simulink library "ECO_TestLibs"  (R2018a)
settings: Solver=ode45  StartTime=0.0  StopTime=10.0  RelTol=1e-3  EnableMultiTasking=on
undefined symbols (not defined in the file or in its folder): h, km
libraries: CoderSF_BSW_Libs x643, $bdroot x217, SF_CanService_Libs x60, simulink x12
(part 3 of 7)

== system ECO_TestLibs/TAF_CAND/Enabled Subsystem ==
  In1 : Inport
  Enable : EnablePort
  "Send CAN Message " : SF_CanService_Libs/Send CAN Message   typeCAN=Connected  channel=CAN_D  mEn=off  msgInfo=TAF_CAN_new  msgIterm=CAN0x7fc  msgItermStore=CAN0x7fc  motoBit=off  flgNoFixed=off  tSample=Task_MDef  modeCode=Parameterless
  Send CAN Message 1 : SF_CanService_Libs/Send CAN Message   typeCAN=Connected  channel=CAN_D  mEn=off  msgInfo=TAF_CAN_new  msgIterm=CAN0x1ffffffc  msgItermStore=CAN0x1ffffffc  motoBit=off  flgNoFixed=off  tSample=Task_MDef  modeCode=Parameterless
  wires:
  In1/1 -> Send CAN Message 1/1, "Send CAN Message "/1

== system ECO_TestLibs/TAF_CAND/Receive CAN Message ==
  Receive CAN Message : CoderSF_BSW_Libs/CAN/Receive CAN Message  channel=CAN_D  txid=hex2dec('100')  extended=off  txlen=8  tasktimeIndex=Task_L1ms
      settings: SourceProductName=EcoCoder Blocks
  Receive CAN Message1 : CoderSF_BSW_Libs/CAN/Receive CAN Message  channel=CAN_D  txid=hex2dec('100')  extended=off  txlen=8  tasktimeIndex=Task_L1ms
      settings: SourceProductName=EcoCoder Blocks
  Receive CAN Message2 : CoderSF_BSW_Libs/CAN/Receive CAN Message  channel=CAN_D  txid=hex2dec('100')  extended=off  txlen=8  tasktimeIndex=Task_L1ms
      settings: SourceProductName=EcoCoder Blocks
  Write Measurement1 : CoderSF_BSW_Libs/Calibration & Measurement/Write Measurement  variable_name=CANDR1_flgAvailable  variable_value=0  variable_type=boolean  numD=1  unitStr=""  descStr=""
      settings: AttributesFormatString=type:%<variable_type> Dimensions:%<numD>  SourceProductName=EcoCoder Blocks
  Write Measurement10 : CoderSF_BSW_Libs/Calibration & Measurement/Write Measurement  variable_name=CANDR2_id  variable_value=0  variable_type=uint32  numD=1  unitStr=""  descStr=""
      settings: AttributesFormatString=type:%<variable_type> Dimensions:%<numD>  SourceProductName=EcoCoder Blocks
  Write Measurement11 : CoderSF_BSW_Libs/Calibration & Measurement/Write Measurement  variable_name=CANDR2_len  variable_value=0  variable_type=uint8  numD=1  unitStr=""  descStr=""
      settings: AttributesFormatString=type:%<variable_type> Dimensions:%<numD>  SourceProductName=EcoCoder Blocks
  Write Measurement12 : CoderSF_BSW_Libs/Calibration & Measurement/Write Measurement  variable_name=CANDR2_data  variable_value=0  variable_type=uint8  numD=8  unitStr=""  descStr=""
      settings: AttributesFormatString=type:%<variable_type> Dimensions:%<numD>  SourceProductName=EcoCoder Blocks
  Write Measurement13 : CoderSF_BSW_Libs/Calibration & Measurement/Write Measurement  variable_name=CANDR3_id  variable_value=0  variable_type=uint32  numD=1  unitStr=""  descStr=""
      settings: AttributesFormatString=type:%<variable_type> Dimensions:%<numD>  SourceProductName=EcoCoder Blocks
  Write Measurement14 : CoderSF_BSW_Libs/Calibration & Measurement/Write Measurement  variable_name=CANDR3_len  variable_value=0  variable_type=uint8  numD=1  unitStr=""  descStr=""
      settings: AttributesFormatString=type:%<variable_type> Dimensions:%<numD>  SourceProductName=EcoCoder Blocks
  Write Measurement15 : CoderSF_BSW_Libs/Calibration & Measurement/Write Measurement  variable_name=CANDR3_data  variable_value=0  variable_type=uint8  numD=8  unitStr=""  descStr=""
      settings: AttributesFormatString=type:%<variable_type> Dimensions:%<numD>  SourceProductName=EcoCoder Blocks
  Write Measurement16 : CoderSF_BSW_Libs/Calibration & Measurement/Write Measurement  variable_name=CANDR3_flgAvailable  variable_value=0  variable_type=boolean  numD=1  unitStr=""  descStr=""
      settings: AttributesFormatString=type:%<variable_type> Dimensions:%<numD>  SourceProductName=EcoCoder Blocks
  Write Measurement17 : CoderSF_BSW_Libs/Calibration & Measurement/Write Measurement  variable_name=CANDR3_flgRemote  variable_value=0  variable_type=boolean  numD=1  unitStr=""  descStr=""
      settings: AttributesFormatString=type:%<variable_type> Dimensions:%<numD>  SourceProductName=EcoCoder Blocks
  Write Measurement18 : CoderSF_BSW_Libs/Calibration & Measurement/Write Measurement  variable_name=CANDR3_flgExtend  variable_value=0  variable_type=boolean  numD=1  unitStr=""  descStr=""
      settings: AttributesFormatString=type:%<variable_type> Dimensions:%<numD>  SourceProductName=EcoCoder Blocks
  Write Measurement19 : CoderSF_BSW_Libs/Calibration & Measurement/Write Measurement  variable_name=CANDR2_flgExtend  variable_value=0  variable_type=boolean  numD=1  unitStr=""  descStr=""
      settings: AttributesFormatString=type:%<variable_type> Dimensions:%<numD>  SourceProductName=EcoCoder Blocks
  Write Measurement3 : CoderSF_BSW_Libs/Calibration & Measurement/Write Measurement  variable_name=CANDR1_flgRemote  variable_value=0  variable_type=boolean  numD=1  unitStr=""  descStr=""
      settings: AttributesFormatString=type:%<variable_type> Dimensions:%<numD>  SourceProductName=EcoCoder Blocks
  Write Measurement4 : CoderSF_BSW_Libs/Calibration & Measurement/Write Measurement  variable_name=CANDR1_flgExtend  variable_value=0  variable_type=boolean  numD=1  unitStr=""  descStr=""
      settings: AttributesFormatString=type:%<variable_type> Dimensions:%<numD>  SourceProductName=EcoCoder Blocks
  Write Measurement5 : CoderSF_BSW_Libs/Calibration & Measurement/Write Measurement  variable_name=CANDR1_id  variable_value=0  variable_type=uint32  numD=1  unitStr=""  descStr=""
      settings: AttributesFormatString=type:%<variable_type> Dimensions:%<numD>  SourceProductName=EcoCoder Blocks
  Write Measurement6 : CoderSF_BSW_Libs/Calibration & Measurement/Write Measurement  variable_name=CANDR1_len  variable_value=0  variable_type=uint8  numD=1  unitStr=""  descStr=""
      settings: AttributesFormatString=type:%<variable_type> Dimensions:%<numD>  SourceProductName=EcoCoder Blocks
  Write Measurement7 : CoderSF_BSW_Libs/Calibration & Measurement/Write Measurement  variable_name=CANDR1_data  variable_value=0  variable_type=uint8  numD=8  unitStr=""  descStr=""
      settings: AttributesFormatString=type:%<variable_type> Dimensions:%<numD>  SourceProductName=EcoCoder Blocks
  Write Measurement8 : CoderSF_BSW_Libs/Calibration & Measurement/Write Measurement  variable_name=CANDR2_flgAvailable  variable_value=0  variable_type=boolean  numD=1  unitStr=""  descStr=""
      settings: AttributesFormatString=type:%<variable_type> Dimensions:%<numD>  SourceProductName=EcoCoder Blocks
  Write Measurement9 : CoderSF_BSW_Libs/Calibration & Measurement/Write Measurement  variable_name=CANDR2_flgRemote  variable_value=0  variable_type=boolean  numD=1  unitStr=""  descStr=""
      settings: AttributesFormatString=type:%<variable_type> Dimensions:%<numD>  SourceProductName=EcoCoder Blocks
  wires:
  Receive CAN Message/1 -> Write Measurement1/1
  Receive CAN Message/2 -> Write Measurement3/1
  Receive CAN Message/3 -> Write Measurement4/1
  Receive CAN Message/4 -> Write Measurement5/1
  Receive CAN Message/5 -> Write Measurement6/1
  Receive CAN Message/6 -> Write Measurement7/1
  Receive CAN Message1/6 -> Write Measurement12/1
  Receive CAN Message1/4 -> Write Measurement10/1
  Receive CAN Message1/1 -> Write Measurement8/1
  Receive CAN Message1/5 -> Write Measurement11/1
  Receive CAN Message1/2 -> Write Measurement9/1
  Receive CAN Message1/3 -> Write Measurement19/1
  Receive CAN Message2/6 -> Write Measurement15/1
  Receive CAN Message2/4 -> Write Measurement13/1
  Receive CAN Message2/1 -> Write Measurement16/1
  Receive CAN Message2/5 -> Write Measurement14/1
  Receive CAN Message2/2 -> Write Measurement17/1
  Receive CAN Message2/3 -> Write Measurement18/1

== system ECO_TestLibs/TAF_CAND/Subsystem ==
  In1 : Inport
  Logical Operator : Logic  AllPortsSameDT=off  OutDataTypeStr=boolean
  Read Calibration : CoderSF_BSW_Libs/Calibration & Measurement/Read Calibration  variable_name=TAF_CAND_flgEnRxResp_val  variable_value=1  variable_type=boolean  variable_min=[]  variable_max=[]  unitStr=""  descStr=""
      settings: AttributesFormatString=value:%<variable_value> type:%<variable_type> max:%<variable_max> Min:%<variable_min>  SourceProductName=EcoCoder Blocks
  Out1 : Outport
  wires:
  Logical Operator/1 -> Out1/1
  Read Calibration/1 -> Logical Operator/1
  In1/1 -> Logical Operator/2

== system ECO_TestLibs/TAF_CANE/Connected ==
  " Override Probe" : CoderSF_BSW_Libs/Calibration & Measurement/ Override Probe  variableName=TAF_CANF_flgEnCANETx  variableValue=1  overrideValue=0  variableDataType=boolean  variableMin=[]  variableMax=[]
      settings: SourceProductName=EcoCoder Blocks
  " Override Probe1" : CoderSF_BSW_Libs/Calibration & Measurement/ Override Probe  variableName=TAF_CAN_flgEnCANETx  variableValue=1  overrideValue=0  variableDataType=boolean  variableMin=[]  variableMax=[]
      settings: SourceProductName=EcoCoder Blocks
  Read CAN Message 4 : SF_CanService_Libs/Read CAN Message  typeCAN=Connected  channel=CAN_E  mEn=off  msgInfo=TAF_CAN_new  msgIterm=CAN0x409x  msgItermStore=CAN0x409x  valid=on  stale=on  motoBit=off  setSignalName=off  defineSignalName=on  prefixSignal='rxCANE'  flgValTest=off  flgNoFixed=off  tSample=Task_L10ms  modeCode=Parameterless
  Read Fixed-Point CAN Message 4 : SF_CanService_Libs/Read Fixed-Point CAN Message   typeCAN=Connected  channel=CAN_E  mEn=off  msgInfo=TAF_CAN_new  msgIterm=CAN0x409  msgItermStore=CAN0x409  valid=on  stale=on  motoBit=off  setSignalName=on  defineSignalName=on  prefixSignal='rxCANE'  flgValTest=off  flgNoFixed=off  tSample=Task_L10ms  modeCode=Parameterless
  Subsystem4 : Subsystem
  Subsystem8 : Subsystem
  Write Measurement12 : CoderSF_BSW_Libs/Calibration & Measurement/Write Measurement  variable_name=TAF_CAN_cntCANERx  variable_value=0  variable_type=uint32  numD=1  unitStr=""  descStr=""
      settings: AttributesFormatString=value:%<variable_value> type:%<variable_type>  SourceProductName=EcoCoder Blocks
  Write Measurement9 : CoderSF_BSW_Libs/Calibration & Measurement/Write Measurement  variable_name=TAF_CANF_cntCANERx  variable_value=0  variable_type=uint32  numD=1  unitStr=""  descStr=""
      settings: AttributesFormatString=value:%<variable_value> type:%<variable_type>  SourceProductName=EcoCoder Blocks
  wires:
  Read Fixed-Point CAN Message 4/1 -> " Override Probe"/1
  Read Fixed-Point CAN Message 4/2 -> Write Measurement9/1
  Read Fixed-Point CAN Message 4/3 -> Subsystem4/1(In1)  "rxCANEByte7"
  Read Fixed-Point CAN Message 4/4 -> Subsystem4/2(In2)  "rxCANEByte6"
  Read Fixed-Point CAN Message 4/5 -> Subsystem4/3(In3)  "rxCANEByte5"
  Read Fixed-Point CAN Message 4/6 -> Subsystem4/4(In4)  "rxCANEByte4"
  Read Fixed-Point CAN Message 4/7 -> Subsystem4/5(In5)  "rxCANEByte3"
  Read Fixed-Point CAN Message 4/8 -> Subsystem4/6(In6)  "rxCANEByte2"
  Read Fixed-Point CAN Message 4/9 -> Subsystem4/7(In7)  "rxCANEByte1"
  Read Fixed-Point CAN Message 4/10 -> Subsystem4/8(In8)  "rxCANEByte0"
  " Override Probe"/1 -> Subsystem4/Enable
  " Override Probe1"/1 -> Subsystem8/Enable
  Read CAN Message 4/10 -> Subsystem8/8(In8)
  Read CAN Message 4/9 -> Subsystem8/7(In7)
  Read CAN Message 4/8 -> Subsystem8/6(In6)
  Read CAN Message 4/7 -> Subsystem8/5(In5)
  Read CAN Message 4/6 -> Subsystem8/4(In4)
  Read CAN Message 4/5 -> Subsystem8/3(In3)
  Read CAN Message 4/4 -> Subsystem8/2(In2)
  Read CAN Message 4/3 -> Subsystem8/1(In1)
  Read CAN Message 4/2 -> Write Measurement12/1
  Read CAN Message 4/1 -> " Override Probe1"/1

== system ECO_TestLibs/TAF_CANE/Disconnected ==
  " Override Probe" : CoderSF_BSW_Libs/Calibration & Measurement/ Override Probe  variableName=TAF_CANF_flgEnCANE2Tx  variableValue=1  overrideValue=0  variableDataType=boolean  variableMin=[]  variableMax=[]
      settings: SourceProductName=EcoCoder Blocks
  " Override Probe1" : CoderSF_BSW_Libs/Calibration & Measurement/ Override Probe  variableName=TAF_CAN_flgEnCANE2Tx  variableValue=1  overrideValue=0  variableDataType=boolean  variableMin=[]  variableMax=[]
      settings: SourceProductName=EcoCoder Blocks
  Read CAN Message 4 : SF_CanService_Libs/Read CAN Message  typeCAN=Disconnected  channel=CAN_E  mEn=off  msgInfo=TAF_CAN_new  msgIterm=CAN0x410x  msgItermStore=CAN0x410x  valid=on  stale=on  motoBit=off  setSignalName=off  defineSignalName=on  prefixSignal='rxCANE'  flgValTest=off  flgNoFixed=off  tSample=Task_L10ms  modeCode=Parameterless
  Read Fixed-Point CAN Message 4 : SF_CanService_Libs/Read Fixed-Point CAN Message   typeCAN=Disconnected  channel=CAN_E  mEn=off  msgInfo=TAF_CAN_new  msgIterm=CAN0x410  msgItermStore=CAN0x410  valid=on  stale=on  motoBit=off  setSignalName=on  defineSignalName=on  prefixSignal='rxCANE2'  flgValTest=off  flgNoFixed=off  tSample=Task_L10ms  modeCode=Parameterless
  Receive CAN Message : CoderSF_BSW_Libs/CAN/Receive CAN Message  channel=CAN_E  txid=hex2dec('410')  extended=off  txlen=8  tasktimeIndex=Task_Inherit
      settings: SourceProductName=EcoCoder Blocks
  Receive CAN Message1 : CoderSF_BSW_Libs/CAN/Receive CAN Message  channel=CAN_E  txid=hex2dec('420')  extended=on  txlen=8  tasktimeIndex=Task_Inherit
      settings: SourceProductName=EcoCoder Blocks
  Subsystem4 : Subsystem
  Subsystem8 : Subsystem
  Write Measurement12 : CoderSF_BSW_Libs/Calibration & Measurement/Write Measurement  variable_name=TAF_CAN_cntCANERx2  variable_value=0  variable_type=uint32  numD=1  unitStr=""  descStr=""
      settings: AttributesFormatString=value:%<variable_value> type:%<variable_type>  SourceProductName=EcoCoder Blocks
  Write Measurement9 : CoderSF_BSW_Libs/Calibration & Measurement/Write Measurement  variable_name=TAF_CANF_cntCANERx2  variable_value=0  variable_type=uint32  numD=1  unitStr=""  descStr=""
      settings: AttributesFormatString=value:%<variable_value> type:%<variable_type>  SourceProductName=EcoCoder Blocks
  wires:
  Receive CAN Message1/5 -> Read CAN Message 4/5
  Receive CAN Message1/3 -> Read CAN Message 4/3
  Receive CAN Message1/6 -> Read CAN Message 4/6
  Receive CAN Message1/4 -> Read CAN Message 4/4
  Receive CAN Message1/1 -> Read CAN Message 4/1
  Receive CAN Message1/2 -> Read CAN Message 4/2
  Receive CAN Message/3 -> Read Fixed-Point CAN Message 4/3
  Receive CAN Message/5 -> Read Fixed-Point CAN Message 4/5
  Receive CAN Message/4 -> Read Fixed-Point CAN Message 4/4
  Receive CAN Message/6 -> Read Fixed-Point CAN Message 4/6
  Receive CAN Message/1 -> Read Fixed-Point CAN Message 4/1
  Receive CAN Message/2 -> Read Fixed-Point CAN Message 4/2
  Read CAN Message 4/1 -> " Override Probe1"/1
  Read CAN Message 4/2 -> Write Measurement12/1
  Read CAN Message 4/3 -> Subsystem8/1(In1)
  Read CAN Message 4/4 -> Subsystem8/2(In2)
  Read CAN Message 4/5 -> Subsystem8/3(In3)
  Read CAN Message 4/6 -> Subsystem8/4(In4)
  Read CAN Message 4/7 -> Subsystem8/5(In5)
  Read CAN Message 4/8 -> Subsystem8/6(In6)
  Read CAN Message 4/9 -> Subsystem8/7(In7)
  Read CAN Message 4/10 -> Subsystem8/8(In8)
  " Override Probe1"/1 -> Subsystem8/Enable
  " Override Probe"/1 -> Subsystem4/Enable
  Read Fixed-Point CAN Message 4/10 -> Subsystem4/8(In8)  "rxCANE2Byte0"
  Read Fixed-Point CAN Message 4/9 -> Subsystem4/7(In7)  "rxCANE2Byte1"
  Read Fixed-Point CAN Message 4/8 -> Subsystem4/6(In6)  "rxCANE2Byte2"
  Read Fixed-Point CAN Message 4/7 -> Subsystem4/5(In5)  "rxCANE2Byte3"
  Read Fixed-Point CAN Message 4/6 -> Subsystem4/4(In4)  "rxCANE2Byte4"
  Read Fixed-Point CAN Message 4/5 -> Subsystem4/3(In3)  "rxCANE2Byte5"
  Read Fixed-Point CAN Message 4/4 -> Subsystem4/2(In2)  "rxCANE2Byte6"
  Read Fixed-Point CAN Message 4/3 -> Subsystem4/1(In1)  "rxCANE2Byte7"
  Read Fixed-Point CAN Message 4/2 -> Write Measurement9/1
  Read Fixed-Point CAN Message 4/1 -> " Override Probe"/1

== system ECO_TestLibs/TAF_CANE/Enabled Subsystem ==
  In1 : Inport
  Enable : EnablePort
  "Send CAN Message " : SF_CanService_Libs/Send CAN Message   typeCAN=Connected  channel=CAN_E  mEn=off  msgInfo=TAF_CAN_new  msgIterm=CAN0x0  msgItermStore=CAN0x0  motoBit=off  flgNoFixed=off  tSample=Task_Inherit  modeCode=Parameterless
  Send CAN Message 1 : SF_CanService_Libs/Send CAN Message   typeCAN=Connected  channel=CAN_E  mEn=off  msgInfo=TAF_CAN_new  msgIterm=CAN0x0x  msgItermStore=CAN0x0x  motoBit=off  flgNoFixed=off  tSample=Task_Inherit  modeCode=Parameterless
  wires:
  In1/1 -> "Send CAN Message "/1, Send CAN Message 1/1

== system ECO_TestLibs/TAF_CANE/Receive CAN Message ==
  Receive CAN Message : CoderSF_BSW_Libs/CAN/Receive CAN Message  channel=CAN_E  txid=hex2dec('100')  extended=off  txlen=8  tasktimeIndex=Task_L1ms
      settings: SourceProductName=EcoCoder Blocks
  Receive CAN Message1 : CoderSF_BSW_Libs/CAN/Receive CAN Message  channel=CAN_E  txid=hex2dec('100')  extended=off  txlen=8  tasktimeIndex=Task_L1ms
      settings: SourceProductName=EcoCoder Blocks
  Receive CAN Message2 : CoderSF_BSW_Libs/CAN/Receive CAN Message  channel=CAN_E  txid=hex2dec('100')  extended=off  txlen=8  tasktimeIndex=Task_L1ms
      settings: SourceProductName=EcoCoder Blocks
  Write Measurement1 : CoderSF_BSW_Libs/Calibration & Measurement/Write Measurement  variable_name=CANER1_flgAvailable  variable_value=0  variable_type=boolean  numD=1  unitStr=""  descStr=""
      settings: AttributesFormatString=type:%<variable_type> Dimensions:%<numD>  SourceProductName=EcoCoder Blocks
  Write Measurement10 : CoderSF_BSW_Libs/Calibration & Measurement/Write Measurement  variable_name=CANER2_id  variable_value=0  variable_type=uint32  numD=1  unitStr=""  descStr=""
      settings: AttributesFormatString=type:%<variable_type> Dimensions:%<numD>  SourceProductName=EcoCoder Blocks
  Write Measurement11 : CoderSF_BSW_Libs/Calibration & Measurement/Write Measurement  variable_name=CANER2_len  variable_value=0  variable_type=uint8  numD=1  unitStr=""  descStr=""
      settings: AttributesFormatString=type:%<variable_type> Dimensions:%<numD>  SourceProductName=EcoCoder Blocks
  Write Measurement12 : CoderSF_BSW_Libs/Calibration & Measurement/Write Measurement  variable_name=CANER2_data  variable_value=0  variable_type=uint8  numD=8  unitStr=""  descStr=""
      settings: AttributesFormatString=type:%<variable_type> Dimensions:%<numD>  SourceProductName=EcoCoder Blocks
  Write Measurement13 : CoderSF_BSW_Libs/Calibration & Measurement/Write Measurement  variable_name=CANER3_id  variable_value=0  variable_type=uint32  numD=1  unitStr=""  descStr=""
      settings: AttributesFormatString=type:%<variable_type> Dimensions:%<numD>  SourceProductName=EcoCoder Blocks
  Write Measurement14 : CoderSF_BSW_Libs/Calibration & Measurement/Write Measurement  variable_name=CANER3_len  variable_value=0  variable_type=uint8  numD=1  unitStr=""  descStr=""
      settings: AttributesFormatString=type:%<variable_type> Dimensions:%<numD>  SourceProductName=EcoCoder Blocks
  Write Measurement15 : CoderSF_BSW_Libs/Calibration & Measurement/Write Measurement  variable_name=CANER3_data  variable_value=0  variable_type=uint8  numD=8  unitStr=""  descStr=""
      settings: AttributesFormatString=type:%<variable_type> Dimensions:%<numD>  SourceProductName=EcoCoder Blocks
  Write Measurement16 : CoderSF_BSW_Libs/Calibration & Measurement/Write Measurement  variable_name=CANER3_flgAvailable  variable_value=0  variable_type=boolean  numD=1  unitStr=""  descStr=""
      settings: AttributesFormatString=type:%<variable_type> Dimensions:%<numD>  SourceProductName=EcoCoder Blocks
  Write Measurement17 : CoderSF_BSW_Libs/Calibration & Measurement/Write Measurement  variable_name=CANER3_flgRemote  variable_value=0  variable_type=boolean  numD=1  unitStr=""  descStr=""
      settings: AttributesFormatString=type:%<variable_type> Dimensions:%<numD>  SourceProductName=EcoCoder Blocks
  Write Measurement18 : CoderSF_BSW_Libs/Calibration & Measurement/Write Measurement  variable_name=CANER3_flgExtend  variable_value=0  variable_type=boolean  numD=1  unitStr=""  descStr=""
      settings: AttributesFormatString=type:%<variable_type> Dimensions:%<numD>  SourceProductName=EcoCoder Blocks
  Write Measurement19 : CoderSF_BSW_Libs/Calibration & Measurement/Write Measurement  variable_name=CANER2_flgExtend  variable_value=0  variable_type=boolean  numD=1  unitStr=""  descStr=""
      settings: AttributesFormatString=type:%<variable_type> Dimensions:%<numD>  SourceProductName=EcoCoder Blocks
  Write Measurement3 : CoderSF_BSW_Libs/Calibration & Measurement/Write Measurement  variable_name=CANER1_flgRemote  variable_value=0  variable_type=boolean  numD=1  unitStr=""  descStr=""
      settings: AttributesFormatString=type:%<variable_type> Dimensions:%<numD>  SourceProductName=EcoCoder Blocks
  Write Measurement4 : CoderSF_BSW_Libs/Calibration & Measurement/Write Measurement  variable_name=CANER1_flgExtend  variable_value=0  variable_type=boolean  numD=1  unitStr=""  descStr=""
      settings: AttributesFormatString=type:%<variable_type> Dimensions:%<numD>  SourceProductName=EcoCoder Blocks
  Write Measurement5 : CoderSF_BSW_Libs/Calibration & Measurement/Write Measurement  variable_name=CANER1_id  variable_value=0  variable_type=uint32  numD=1  unitStr=""  descStr=""
      settings: AttributesFormatString=type:%<variable_type> Dimensions:%<numD>  SourceProductName=EcoCoder Blocks
  Write Measurement6 : CoderSF_BSW_Libs/Calibration & Measurement/Write Measurement  variable_name=CANER1_len  variable_value=0  variable_type=uint8  numD=1  unitStr=""  descStr=""
      settings: AttributesFormatString=type:%<variable_type> Dimensions:%<numD>  SourceProductName=EcoCoder Blocks
  Write Measurement7 : CoderSF_BSW_Libs/Calibration & Measurement/Write Measurement  variable_name=CANER1_data  variable_value=0  variable_type=uint8  numD=8  unitStr=""  descStr=""
      settings: AttributesFormatString=type:%<variable_type> Dimensions:%<numD>  SourceProductName=EcoCoder Blocks
  Write Measurement8 : CoderSF_BSW_Libs/Calibration & Measurement/Write Measurement  variable_name=CANER2_flgAvailable  variable_value=0  variable_type=boolean  numD=1  unitStr=""  descStr=""
      settings: AttributesFormatString=type:%<variable_type> Dimensions:%<numD>  SourceProductName=EcoCoder Blocks
  Write Measurement9 : CoderSF_BSW_Libs/Calibration & Measurement/Write Measurement  variable_name=CANER2_flgRemote  variable_value=0  variable_type=boolean  numD=1  unitStr=""  descStr=""
      settings: AttributesFormatString=type:%<variable_type> Dimensions:%<numD>  SourceProductName=EcoCoder Blocks
  wires:
  Receive CAN Message/1 -> Write Measurement1/1
  Receive CAN Message/2 -> Write Measurement3/1
  Receive CAN Message/3 -> Write Measurement4/1
  Receive CAN Message/4 -> Write Measurement5/1
  Receive CAN Message/5 -> Write Measurement6/1
  Receive CAN Message/6 -> Write Measurement7/1
  Receive CAN Message1/6 -> Write Measurement12/1
  Receive CAN Message1/4 -> Write Measurement10/1
  Receive CAN Message1/1 -> Write Measurement8/1
  Receive CAN Message1/5 -> Write Measurement11/1
  Receive CAN Message1/2 -> Write Measurement9/1
  Receive CAN Message1/3 -> Write Measurement19/1
  Receive CAN Message2/6 -> Write Measurement15/1
  Receive CAN Message2/4 -> Write Measurement13/1
  Receive CAN Message2/1 -> Write Measurement16/1
  Receive CAN Message2/5 -> Write Measurement14/1
  Receive CAN Message2/2 -> Write Measurement17/1
  Receive CAN Message2/3 -> Write Measurement18/1

== system ECO_TestLibs/TAF_CANE/Subsystem ==
  In1 : Inport
  Logical Operator : Logic  AllPortsSameDT=off  OutDataTypeStr=boolean
  Read Calibration : CoderSF_BSW_Libs/Calibration & Measurement/Read Calibration  variable_name=TAF_CANE_flgEnRxResp_val  variable_value=1  variable_type=boolean  variable_min=[]  variable_max=[]  unitStr=""  descStr=""
      settings: AttributesFormatString=value:%<variable_value> type:%<variable_type> max:%<variable_max> Min:%<variable_min>  SourceProductName=EcoCoder Blocks
  Out1 : Outport
  wires:
  Logical Operator/1 -> Out1/1
  Read Calibration/1 -> Logical Operator/1
  In1/1 -> Logical Operator/2

== system ECO_TestLibs/TAF_CANF/Connected ==
  " Override Probe" : CoderSF_BSW_Libs/Calibration & Measurement/ Override Probe  variableName=TAF_CANF_flgEnCANFTx  variableValue=1  overrideValue=0  variableDataType=boolean  variableMin=[]  variableMax=[]
      settings: SourceProductName=EcoCoder Blocks
  " Override Probe1" : CoderSF_BSW_Libs/Calibration & Measurement/ Override Probe  variableName=TAF_CAN_flgEnCANFTx  variableValue=1  overrideValue=0  variableDataType=boolean  variableMin=[]  variableMax=[]
      settings: SourceProductName=EcoCoder Blocks
  Read CAN Message 4 : SF_CanService_Libs/Read CAN Message  typeCAN=Connected  channel=CAN_F  mEn=off  msgInfo=TAF_CAN_new  msgIterm=CAN0x409x  msgItermStore=CAN0x409x  valid=on  stale=on  motoBit=off  setSignalName=off  defineSignalName=on  prefixSignal='rxCANE'  flgValTest=off  flgNoFixed=off  tSample=Task_L10ms  modeCode=Parameterless
  Read Fixed-Point CAN Message 4 : SF_CanService_Libs/Read Fixed-Point CAN Message   typeCAN=Connected  channel=CAN_F  mEn=off  msgInfo=TAF_CAN_new  msgIterm=CAN0x409  msgItermStore=CAN0x409  valid=on  stale=on  motoBit=off  setSignalName=on  defineSignalName=on  prefixSignal='rxCANF'  flgValTest=off  flgNoFixed=off  tSample=Task_L10ms  modeCode=Parameterless
  Subsystem4 : Subsystem
  Subsystem8 : Subsystem
  Write Measurement12 : CoderSF_BSW_Libs/Calibration & Measurement/Write Measurement  variable_name=TAF_CAN_cntCANFRx  variable_value=0  variable_type=uint32  numD=1  unitStr=""  descStr=""
      settings: AttributesFormatString=value:%<variable_value> type:%<variable_type>  SourceProductName=EcoCoder Blocks
  Write Measurement9 : CoderSF_BSW_Libs/Calibration & Measurement/Write Measurement  variable_name=TAF_CANF_cntCANFRx  variable_value=0  variable_type=uint32  numD=1  unitStr=""  descStr=""
      settings: AttributesFormatString=value:%<variable_value> type:%<variable_type>  SourceProductName=EcoCoder Blocks
  wires:
  Read CAN Message 4/1 -> " Override Probe1"/1
  Read CAN Message 4/2 -> Write Measurement12/1
  Read CAN Message 4/3 -> Subsystem8/1(In1)
  Read CAN Message 4/4 -> Subsystem8/2(In2)
  Read CAN Message 4/5 -> Subsystem8/3(In3)
  Read CAN Message 4/6 -> Subsystem8/4(In4)
  Read CAN Message 4/7 -> Subsystem8/5(In5)
  Read CAN Message 4/8 -> Subsystem8/6(In6)
  Read CAN Message 4/9 -> Subsystem8/7(In7)
  Read CAN Message 4/10 -> Subsystem8/8(In8)
  " Override Probe1"/1 -> Subsystem8/Enable
  " Override Probe"/1 -> Subsystem4/Enable
  Read Fixed-Point CAN Message 4/10 -> Subsystem4/8(In8)  "rxCANFByte0"
  Read Fixed-Point CAN Message 4/9 -> Subsystem4/7(In7)  "rxCANFByte1"
  Read Fixed-Point CAN Message 4/8 -> Subsystem4/6(In6)  "rxCANFByte2"
  Read Fixed-Point CAN Message 4/7 -> Subsystem4/5(In5)  "rxCANFByte3"
  Read Fixed-Point CAN Message 4/6 -> Subsystem4/4(In4)  "rxCANFByte4"
  Read Fixed-Point CAN Message 4/5 -> Subsystem4/3(In3)  "rxCANFByte5"
  Read Fixed-Point CAN Message 4/4 -> Subsystem4/2(In2)  "rxCANFByte6"
  Read Fixed-Point CAN Message 4/3 -> Subsystem4/1(In1)  "rxCANFByte7"
  Read Fixed-Point CAN Message 4/2 -> Write Measurement9/1
  Read Fixed-Point CAN Message 4/1 -> " Override Probe"/1

== system ECO_TestLibs/TAF_CANF/Disconnected ==
  " Override Probe" : CoderSF_BSW_Libs/Calibration & Measurement/ Override Probe  variableName=TAF_CANF_flgEnCANF2Tx  variableValue=1  overrideValue=0  variableDataType=boolean  variableMin=[]  variableMax=[]
      settings: SourceProductName=EcoCoder Blocks
  " Override Probe1" : CoderSF_BSW_Libs/Calibration & Measurement/ Override Probe  variableName=TAF_CAN_flgEnCANF2Tx  variableValue=1  overrideValue=0  variableDataType=boolean  variableMin=[]  variableMax=[]
      settings: SourceProductName=EcoCoder Blocks
  Read CAN Message 4 : SF_CanService_Libs/Read CAN Message  typeCAN=Disconnected  channel=CAN_F  mEn=off  msgInfo=TAF_CAN_new  msgIterm=CAN0x410x  msgItermStore=CAN0x410x  valid=on  stale=on  motoBit=off  setSignalName=off  defineSignalName=on  prefixSignal='rxCANE'  flgValTest=off  flgNoFixed=off  tSample=Task_L10ms  modeCode=Parameterless
  Read Fixed-Point CAN Message 4 : SF_CanService_Libs/Read Fixed-Point CAN Message   typeCAN=Disconnected  channel=CAN_F  mEn=off  msgInfo=TAF_CAN_new  msgIterm=CAN0x410  msgItermStore=CAN0x410  valid=on  stale=on  motoBit=off  setSignalName=on  defineSignalName=on  prefixSignal='rxCANF2'  flgValTest=off  flgNoFixed=off  tSample=Task_L10ms  modeCode=Parameterless
  Receive CAN Message : CoderSF_BSW_Libs/CAN/Receive CAN Message  channel=CAN_F  txid=hex2dec('410')  extended=off  txlen=8  tasktimeIndex=Task_Inherit
      settings: SourceProductName=EcoCoder Blocks
  Receive CAN Message1 : CoderSF_BSW_Libs/CAN/Receive CAN Message  channel=CAN_F  txid=hex2dec('420')  extended=on  txlen=8  tasktimeIndex=Task_Inherit
      settings: SourceProductName=EcoCoder Blocks
  Subsystem4 : Subsystem
  Subsystem8 : Subsystem
  Write Measurement12 : CoderSF_BSW_Libs/Calibration & Measurement/Write Measurement  variable_name=TAF_CAN_cntCANFRx2  variable_value=0  variable_type=uint32  numD=1  unitStr=""  descStr=""
      settings: AttributesFormatString=value:%<variable_value> type:%<variable_type>  SourceProductName=EcoCoder Blocks
  Write Measurement9 : CoderSF_BSW_Libs/Calibration & Measurement/Write Measurement  variable_name=TAF_CANF_cntCANFRx2  variable_value=0  variable_type=uint32  numD=1  unitStr=""  descStr=""
      settings: AttributesFormatString=value:%<variable_value> type:%<variable_type>  SourceProductName=EcoCoder Blocks
  wires:
  Read Fixed-Point CAN Message 4/1 -> " Override Probe"/1
  Read Fixed-Point CAN Message 4/2 -> Write Measurement9/1
  Read Fixed-Point CAN Message 4/3 -> Subsystem4/1(In1)  "rxCANF2Byte7"
  Read Fixed-Point CAN Message 4/4 -> Subsystem4/2(In2)  "rxCANF2Byte6"
  Read Fixed-Point CAN Message 4/5 -> Subsystem4/3(In3)  "rxCANF2Byte5"
  Read Fixed-Point CAN Message 4/6 -> Subsystem4/4(In4)  "rxCANF2Byte4"
  Read Fixed-Point CAN Message 4/7 -> Subsystem4/5(In5)  "rxCANF2Byte3"
  Read Fixed-Point CAN Message 4/8 -> Subsystem4/6(In6)  "rxCANF2Byte2"
  Read Fixed-Point CAN Message 4/9 -> Subsystem4/7(In7)  "rxCANF2Byte1"
  Read Fixed-Point CAN Message 4/10 -> Subsystem4/8(In8)  "rxCANF2Byte0"
  " Override Probe"/1 -> Subsystem4/Enable
  " Override Probe1"/1 -> Subsystem8/Enable
  Read CAN Message 4/10 -> Subsystem8/8(In8)
  Read CAN Message 4/9 -> Subsystem8/7(In7)
  Read CAN Message 4/8 -> Subsystem8/6(In6)
  Read CAN Message 4/7 -> Subsystem8/5(In5)
  Read CAN Message 4/6 -> Subsystem8/4(In4)
  Read CAN Message 4/5 -> Subsystem8/3(In3)
  Read CAN Message 4/4 -> Subsystem8/2(In2)
  Read CAN Message 4/3 -> Subsystem8/1(In1)
  Read CAN Message 4/2 -> Write Measurement12/1
  Read CAN Message 4/1 -> " Override Probe1"/1
  Receive CAN Message/2 -> Read Fixed-Point CAN Message 4/2
  Receive CAN Message/1 -> Read Fixed-Point CAN Message 4/1
  Receive CAN Message/6 -> Read Fixed-Point CAN Message 4/6
  Receive CAN Message/4 -> Read Fixed-Point CAN Message 4/4
  Receive CAN Message/5 -> Read Fixed-Point CAN Message 4/5
  Receive CAN Message/3 -> Read Fixed-Point CAN Message 4/3
  Receive CAN Message1/2 -> Read CAN Message 4/2
  Receive CAN Message1/1 -> Read CAN Message 4/1
  Receive CAN Message1/4 -> Read CAN Message 4/4
  Receive CAN Message1/6 -> Read CAN Message 4/6
  Receive CAN Message1/3 -> Read CAN Message 4/3
  Receive CAN Message1/5 -> Read CAN Message 4/5

== system ECO_TestLibs/TAF_CANF/Enabled Subsystem ==
  In1 : Inport
  Enable : EnablePort
  "Send CAN Message " : SF_CanService_Libs/Send CAN Message   typeCAN=Connected  channel=CAN_F  mEn=off  msgInfo=TAF_CAN_new  msgIterm=CAN0x0  msgItermStore=CAN0x0  motoBit=off  flgNoFixed=off  tSample=Task_MDef  modeCode=Parameterless
  Send CAN Message 1 : SF_CanService_Libs/Send CAN Message   typeCAN=Connected  channel=CAN_F  mEn=off  msgInfo=TAF_CAN_new  msgIterm=CAN0x0x  msgItermStore=CAN0x0x  motoBit=off  flgNoFixed=off  tSample=Task_MDef  modeCode=Parameterless
  wires:
  In1/1 -> Send CAN Message 1/1, "Send CAN Message "/1

== system ECO_TestLibs/TAF_CANF/Receive CAN Message ==
  Receive CAN Message : CoderSF_BSW_Libs/CAN/Receive CAN Message  channel=CAN_F  txid=hex2dec('100')  extended=off  txlen=8  tasktimeIndex=Task_L1ms
      settings: SourceProductName=EcoCoder Blocks
  Receive CAN Message1 : CoderSF_BSW_Libs/CAN/Receive CAN Message  channel=CAN_F  txid=hex2dec('100')  extended=off  txlen=8  tasktimeIndex=Task_L1ms
      settings: SourceProductName=EcoCoder Blocks
  Receive CAN Message2 : CoderSF_BSW_Libs/CAN/Receive CAN Message  channel=CAN_F  txid=hex2dec('100')  extended=off  txlen=8  tasktimeIndex=Task_L1ms
      settings: SourceProductName=EcoCoder Blocks
  Write Measurement1 : CoderSF_BSW_Libs/Calibration & Measurement/Write Measurement  variable_name=CANFR1_flgAvailable  variable_value=0  variable_type=boolean  numD=1  unitStr=""  descStr=""
      settings: AttributesFormatString=type:%<variable_type> Dimensions:%<numD>  SourceProductName=EcoCoder Blocks
  Write Measurement10 : CoderSF_BSW_Libs/Calibration & Measurement/Write Measurement  variable_name=CANFR2_id  variable_value=0  variable_type=uint32  numD=1  unitStr=""  descStr=""
      settings: AttributesFormatString=type:%<variable_type> Dimensions:%<numD>  SourceProductName=EcoCoder Blocks
  Write Measurement11 : CoderSF_BSW_Libs/Calibration & Measurement/Write Measurement  variable_name=CANFR2_len  variable_value=0  variable_type=uint8  numD=1  unitStr=""  descStr=""
      settings: AttributesFormatString=type:%<variable_type> Dimensions:%<numD>  SourceProductName=EcoCoder Blocks
  Write Measurement12 : CoderSF_BSW_Libs/Calibration & Measurement/Write Measurement  variable_name=CANFR2_data  variable_value=0  variable_type=uint8  numD=8  unitStr=""  descStr=""
      settings: AttributesFormatString=type:%<variable_type> Dimensions:%<numD>  SourceProductName=EcoCoder Blocks
  Write Measurement13 : CoderSF_BSW_Libs/Calibration & Measurement/Write Measurement  variable_name=CANFR3_id  variable_value=0  variable_type=uint32  numD=1  unitStr=""  descStr=""
      settings: AttributesFormatString=type:%<variable_type> Dimensions:%<numD>  SourceProductName=EcoCoder Blocks
  Write Measurement14 : CoderSF_BSW_Libs/Calibration & Measurement/Write Measurement  variable_name=CANFR3_len  variable_value=0  variable_type=uint8  numD=1  unitStr=""  descStr=""
      settings: AttributesFormatString=type:%<variable_type> Dimensions:%<numD>  SourceProductName=EcoCoder Blocks
  Write Measurement15 : CoderSF_BSW_Libs/Calibration & Measurement/Write Measurement  variable_name=CANFR3_data  variable_value=0  variable_type=uint8  numD=8  unitStr=""  descStr=""
      settings: AttributesFormatString=type:%<variable_type> Dimensions:%<numD>  SourceProductName=EcoCoder Blocks
  Write Measurement16 : CoderSF_BSW_Libs/Calibration & Measurement/Write Measurement  variable_name=CANFR3_flgAvailable  variable_value=0  variable_type=boolean  numD=1  unitStr=""  descStr=""
      settings: AttributesFormatString=type:%<variable_type> Dimensions:%<numD>  SourceProductName=EcoCoder Blocks
  Write Measurement17 : CoderSF_BSW_Libs/Calibration & Measurement/Write Measurement  variable_name=CANFR3_flgRemote  variable_value=0  variable_type=boolean  numD=1  unitStr=""  descStr=""
      settings: AttributesFormatString=type:%<variable_type> Dimensions:%<numD>  SourceProductName=EcoCoder Blocks
  Write Measurement18 : CoderSF_BSW_Libs/Calibration & Measurement/Write Measurement  variable_name=CANFR3_flgExtend  variable_value=0  variable_type=boolean  numD=1  unitStr=""  descStr=""
      settings: AttributesFormatString=type:%<variable_type> Dimensions:%<numD>  SourceProductName=EcoCoder Blocks
  Write Measurement19 : CoderSF_BSW_Libs/Calibration & Measurement/Write Measurement  variable_name=CANFR2_flgExtend  variable_value=0  variable_type=boolean  numD=1  unitStr=""  descStr=""
      settings: AttributesFormatString=type:%<variable_type> Dimensions:%<numD>  SourceProductName=EcoCoder Blocks
  Write Measurement3 : CoderSF_BSW_Libs/Calibration & Measurement/Write Measurement  variable_name=CANFR1_flgRemote  variable_value=0  variable_type=boolean  numD=1  unitStr=""  descStr=""
      settings: AttributesFormatString=type:%<variable_type> Dimensions:%<numD>  SourceProductName=EcoCoder Blocks
  Write Measurement4 : CoderSF_BSW_Libs/Calibration & Measurement/Write Measurement  variable_name=CANFR1_flgExtend  variable_value=0  variable_type=boolean  numD=1  unitStr=""  descStr=""
      settings: AttributesFormatString=type:%<variable_type> Dimensions:%<numD>  SourceProductName=EcoCoder Blocks
  Write Measurement5 : CoderSF_BSW_Libs/Calibration & Measurement/Write Measurement  variable_name=CANFR1_id  variable_value=0  variable_type=uint32  numD=1  unitStr=""  descStr=""
      settings: AttributesFormatString=type:%<variable_type> Dimensions:%<numD>  SourceProductName=EcoCoder Blocks
  Write Measurement6 : CoderSF_BSW_Libs/Calibration & Measurement/Write Measurement  variable_name=CANFR1_len  variable_value=0  variable_type=uint8  numD=1  unitStr=""  descStr=""
      settings: AttributesFormatString=type:%<variable_type> Dimensions:%<numD>  SourceProductName=EcoCoder Blocks
  Write Measurement7 : CoderSF_BSW_Libs/Calibration & Measurement/Write Measurement  variable_name=CANFR1_data  variable_value=0  variable_type=uint8  numD=8  unitStr=""  descStr=""
      settings: AttributesFormatString=type:%<variable_type> Dimensions:%<numD>  SourceProductName=EcoCoder Blocks
  Write Measurement8 : CoderSF_BSW_Libs/Calibration & Measurement/Write Measurement  variable_name=CANFR2_flgAvailable  variable_value=0  variable_type=boolean  numD=1  unitStr=""  descStr=""
      settings: AttributesFormatString=type:%<variable_type> Dimensions:%<numD>  SourceProductName=EcoCoder Blocks
  Write Measurement9 : CoderSF_BSW_Libs/Calibration & Measurement/Write Measurement  variable_name=CANFR2_flgRemote  variable_value=0  variable_type=boolean  numD=1  unitStr=""  descStr=""
      settings: AttributesFormatString=type:%<variable_type> Dimensions:%<numD>  SourceProductName=EcoCoder Blocks
  wires:
  Receive CAN Message/1 -> Write Measurement1/1
  Receive CAN Message/2 -> Write Measurement3/1
  Receive CAN Message/3 -> Write Measurement4/1
  Receive CAN Message/4 -> Write Measurement5/1
  Receive CAN Message/5 -> Write Measurement6/1
  Receive CAN Message/6 -> Write Measurement7/1
  Receive CAN Message1/6 -> Write Measurement12/1
  Receive CAN Message1/4 -> Write Measurement10/1
  Receive CAN Message1/1 -> Write Measurement8/1
  Receive CAN Message1/5 -> Write Measurement11/1
  Receive CAN Message1/2 -> Write Measurement9/1
  Receive CAN Message1/3 -> Write Measurement19/1
  Receive CAN Message2/6 -> Write Measurement15/1
  Receive CAN Message2/4 -> Write Measurement13/1
  Receive CAN Message2/1 -> Write Measurement16/1
  Receive CAN Message2/5 -> Write Measurement14/1
  Receive CAN Message2/2 -> Write Measurement17/1
  Receive CAN Message2/3 -> Write Measurement18/1

== system ECO_TestLibs/TAF_CANF/Subsystem ==
  In1 : Inport
  Logical Operator : Logic  AllPortsSameDT=off  OutDataTypeStr=boolean
  Read Calibration : CoderSF_BSW_Libs/Calibration & Measurement/Read Calibration  variable_name=TAF_CANF_flgEnRxResp_val  variable_value=1  variable_type=boolean  variable_min=[]  variable_max=[]  unitStr=""  descStr=""
      settings: AttributesFormatString=value:%<variable_value> type:%<variable_type> max:%<variable_max> Min:%<variable_min>  SourceProductName=EcoCoder Blocks
  Out1 : Outport
  wires:
  Logical Operator/1 -> Out1/1
  Read Calibration/1 -> Logical Operator/1
  In1/1 -> Logical Operator/2

== system ECO_TestLibs/TAF_CM/F Calibration Data Check ==
  function : TriggerPort  TriggerType=function-call  VariantControl=(inherit)
  Constant : Constant  Value=[5 4 5 5 4 4 4 4]  OutDataTypeStr=uint8  SampleTime=-1
  Constant1 : Constant  Value=[5 4 5 5 4 4 4 4]  OutDataTypeStr=uint8  SampleTime=-1
  Constant2 : Constant  Value=[5 4 5 5 4 4 4 4]  OutDataTypeStr=uint8  SampleTime=-1
  Send CAN Data : CoderSF_BSW_Libs/CAN/Send CAN Data  channel=CAN_A  txlen=2  txid=hex2dec('554')  frametype=Extended(29-bit ID)  showerror=off
      settings: SourceProductName=EcoCoder Blocks
  Send CAN Data1 : CoderSF_BSW_Libs/CAN/Send CAN Data  channel=CAN_B  txlen=2  txid=hex2dec('555')  frametype=Extended(29-bit ID)  showerror=off
      settings: SourceProductName=EcoCoder Blocks
  Send CAN Data2 : CoderSF_BSW_Libs/CAN/Send CAN Data  channel=CAN_C  txlen=2  txid=hex2dec('556')  frametype=Extended(29-bit ID)  showerror=off
      settings: SourceProductName=EcoCoder Blocks
  wires:
  Constant/1 -> Send CAN Data/1
  Constant1/1 -> Send CAN Data1/1
  Constant2/1 -> Send CAN Data2/1
